simulink model "TwoDSim"  (R2021b)
settings: Solver=VariableStepAuto  StartTime=0.0  StopTime=5  RelTol=1e-3
undefined symbols (not defined in the file): Dterm, Iterm, Pterm
libraries: simulink_extras x5, simulink x1, slpidlib x1
settings Model: Creator=Andres  LastModifiedBy=Andres
settings SolverCC: ZeroCrossAlgorithm=Adaptive
settings DebuggingCC: IgnoredZcDiagnostic=none

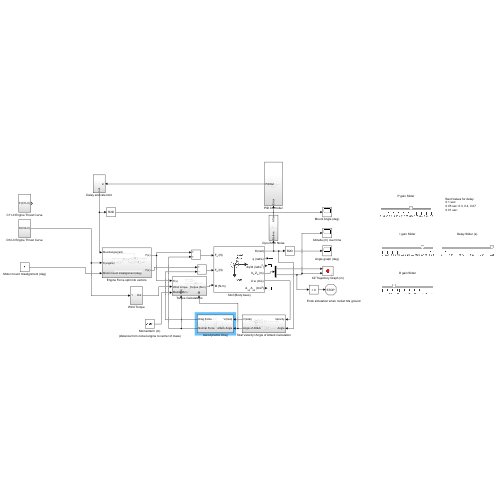
[thumbnail: Simulink's stored preview of the top-level diagram]
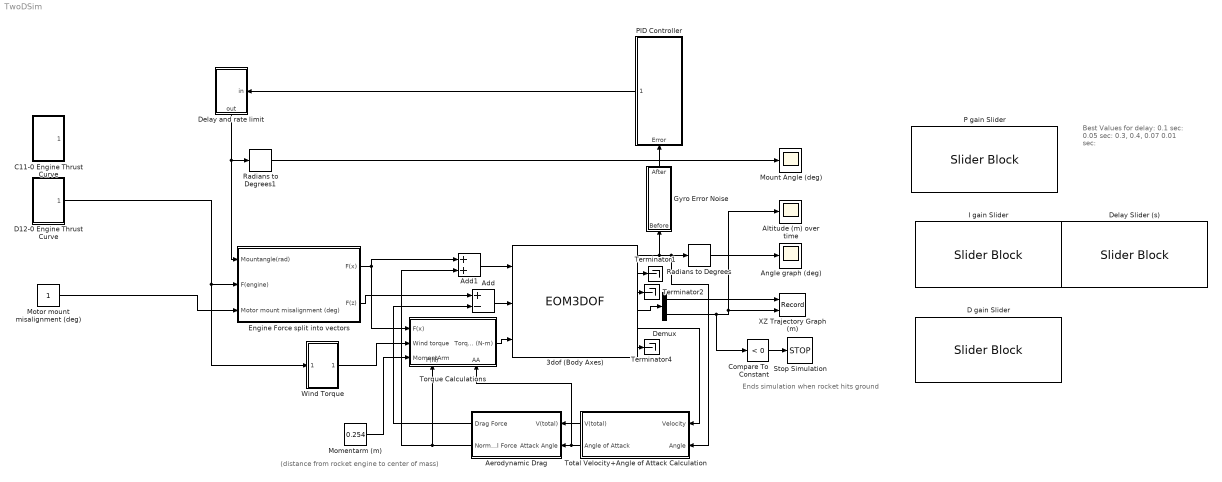
== system TwoDSim ==
  note: Ends simulation when rocket hits ground
  note: (distance from rocket engine to center of mass)
  note: Best Values for delay:
      | 0.1 sec:
      | 0.05 sec: 0.3, 0.4, 0.07
      | 0.01 sec:
  3dof (Body Axes) : EOM3DOF  v_ini=0.00000000000000000001  pos_ini=[0 0.1]  mass=0.688  Iyy=0.012545  g=-9.81
  Add : Sum  Inputs=+-
  Add1 : Sum
  Aerodynamic Drag : Subsystem
  Altitude (m) over time : Scope
  Angle graph (deg) : Scope
  C11-0 Engine Thrust Curve : Subsystem
  Compare To Constant : simulink/Logic and Bit Operations/Compare To Constant  relop=<  const=0  OutDataTypeStr=boolean
  D gain Slider : SliderBlock  LabelPosition=Hide  ScaleMax=0.3
  D12-0 Engine Thrust Curve : Subsystem
  Delay Slider (s) : SliderBlock  LabelPosition=Hide  ScaleMax=0.05  TickInterval=0.01
  Delay and rate limit : Subsystem
      settings: PortSchema="{\"entries\":[{\"content\":{\"sides\":[{\"content\":{\"connectorIds\":[\"In1\"]},\"type\":\"ConnectorPlacement.EquallySpacedRectSide\",\"uuid\":\"7f945310-91d5-4a5b-a152-cb378cea97e0\"},{\"content\":{\"connectorIds\":[],\"side\":\"RIGHT\"},\"type\":\"ConnectorPlacement.EquallySpacedRectSide\",\"uuid\":\"570eb395-808b-402d-8169-834796957515\"},{\"content\":{\"connectorIds\":[],\"side\":\"TOP\"},\"type\":\"ConnectorPlacement.EquallySpacedRectSide\",\"uuid\":\"f414d9f5-06db-41f9-9870-e73b040f5e14\"},{\"content\":{\"connectorIds\":[\"Out1\"],\"side\":\"BOTTOM\"},\"type\":\"ConnectorPlacement.EquallySpacedRectSide\",\"uuid\":\"dd3ad95d-53d5-4309-a4ef-7403eee50954\"}]},\"type\":\"ConnectorPlacement.EquallySpacedConnector\",\"uuid\":\"16f64462-feef-497e-ac9f-2db815891e61\"}],\"packageUris\":[\"http://schema.mathworks.com/mf0/Connector/R2020b\"],\"version\":\"1.0\"}"
  Demux : Demux  Outputs=2
  Engine Force split into vectors : Subsystem
  Gyro Error Noise : Subsystem
      settings: PortSchema="{\"entries\":[{\"content\":{\"sides\":[{\"content\":{\"connectorIds\":[]},\"type\":\"ConnectorPlacement.EquallySpacedRectSide\",\"uuid\":\"db613b74-a95a-4e78-b0b5-852c38ce090d\"},{\"content\":{\"connectorIds\":[],\"side\":\"RIGHT\"},\"type\":\"ConnectorPlacement.EquallySpacedRectSide\",\"uuid\":\"8ff7bb38-cc09-4562-ae4b-2277c61965ca\"},{\"content\":{\"connectorIds\":[\"Out1\"],\"side\":\"TOP\"},\"type\":\"ConnectorPlacement.EquallySpacedRectSide\",\"uuid\":\"fa7b536e-f18b-43ee-b35a-7562f98f0dcc\"},{\"content\":{\"connectorIds\":[\"In1\"],\"side\":\"BOTTOM\"},\"type\":\"ConnectorPlacement.EquallySpacedRectSide\",\"uuid\":\"dd72ef68-23e3-4e8c-8031-36f0d8372741\"}]},\"type\":\"ConnectorPlacement.EquallySpacedConnector\",\"uuid\":\"56970b38-3c02-4837-94fb-dc8b3090c774\"}],\"packageUris\":[\"http://schema.mathworks.com/mf0/Connector/R2020b\"],\"version\":\"1.0\"}"
  I gain Slider : SliderBlock  LabelPosition=Hide  ScaleMax=0.5
  Momentarm (m) : Constant  Value=0.254
  Motor mount misalignment (deg) : Constant
  Mount Angle (deg) : Scope
  P gain Slider : SliderBlock  LabelPosition=Hide  ScaleMax=0.5
  PID Controller : Subsystem
      settings: PortSchema="{\"entries\":[{\"content\":{\"sides\":[{\"content\":{\"connectorIds\":[\"Out1\"]},\"type\":\"ConnectorPlacement.EquallySpacedRectSide\",\"uuid\":\"3056940d-b626-4ad3-aea6-cbabeac63329\"},{\"content\":{\"connectorIds\":[],\"side\":\"RIGHT\"},\"type\":\"ConnectorPlacement.EquallySpacedRectSide\",\"uuid\":\"0510cd9b-8fa4-4f8a-80ec-38231d972233\"},{\"content\":{\"connectorIds\":[],\"side\":\"TOP\"},\"type\":\"ConnectorPlacement.EquallySpacedRectSide\",\"uuid\":\"9c9a70ab-b090-41d6-ac7a-a7598bc3d7a5\"},{\"content\":{\"connectorIds\":[\"In1\"],\"side\":\"BOTTOM\"},\"type\":\"ConnectorPlacement.EquallySpacedRectSide\",\"uuid\":\"76047b82-5909-4180-a207-d443029300af\"}]},\"type\":\"ConnectorPlacement.EquallySpacedConnector\",\"uuid\":\"ba61792f-c506-461f-9738-365393edbd5c\"}],\"packageUris\":[\"http://schema.mathworks.com/mf0/Connector/R2020b\"],\"version\":\"1.0\"}"
  Radians to Degrees : simulink_extras/Transformations/Radians to Degrees
  Radians to Degrees1 : simulink_extras/Transformations/Radians to Degrees
  Stop Simulation : Stop
  Terminator1 : Terminator
  Terminator2 : Terminator
  Terminator4 : Terminator
  Torque Calculations : Subsystem
      settings: PortSchema="{\"entries\":[{\"content\":{\"sides\":[{\"content\":{\"connectorIds\":[\"In1\",\"In2\",\"In3\"]},\"type\":\"ConnectorPlacement.EquallySpacedRectSide\",\"uuid\":\"46c9bf12-68cd-4f09-8bad-0e00413da724\"},{\"content\":{\"connectorIds\":[\"Out1\"],\"side\":\"RIGHT\"},\"type\":\"ConnectorPlacement.EquallySpacedRectSide\",\"uuid\":\"5cb401ed-1243-45d0-bdc5-af7640ec82b5\"},{\"content\":{\"connectorIds\":[],\"side\":\"TOP\"},\"type\":\"ConnectorPlacement.EquallySpacedRectSide\",\"uuid\":\"5f043d3f-b6cd-41df-bbf2-4ec5056a4b50\"},{\"content\":{\"connectorIds\":[\"In4\",\"In5\"],\"side\":\"BOTTOM\"},\"type\":\"ConnectorPlacement.EquallySpacedRectSide\",\"uuid\":\"42e4a957-daef-4922-8ac0-104dea8142f2\"}]},\"type\":\"ConnectorPlacement.EquallySpacedConnector\",\"uuid\":\"e504a0e6-5ad1-4450-ab64-4c7c7eb6b0a6\"}],\"packageUris\":[\"http://schema.mathworks.com/mf0/Connector/R2020b\"],\"version\":\"1.0\"}"
  Total Velocity+Angle of Attack Calculation : Subsystem
  Wind Torque : Subsystem
  XZ Trajectory Graph (m) : Record  FileSettingsInternal="{\"entries\":[{\"content\":{\"excelSettings\":{\"content\":{},\"type\":\"Streamout.ExcelSettings\"}},\"type\":\"Streamout.FileSettingStorage\",\"uuid\":\"bb20e1d7-6d9a-4e8f-a0b6-b3d1b4dfe27c\"}],\"packageUris\":[\"http://schema.mathworks.com/mf0/streamout_blocks/R2020a\"],\"version\":\"1.0\"}"  Layout=[1 1]  SignalsInternal="{\"entries\":[{\"content\":{\"signals\":[{\"content\":{\"blockPath\":[\"TwoDSim/XZ Trajectory Graph (m)\"],\"channel\":[],\"dimensions\":[1],\"domain\":\"TwoDSim/XZ Trajectory Graph (m)\",\"lineColor\":\"#fe330a\",\"plots\":[1],\"port\":1,\"sid\":[\"\"],\"signalID\":2931,\"signalName\":\"Demux:1\"},\"type\":\"RecordBlkView.Signal\",\"uuid\":\"c85508b4-ab53-4732-8bef-55b80f18123d\"},{\"content\":{\"blockPath\":[\"TwoDSim/XZ Trajectory Graph (m)\"],\"channel\":[],\"dimensions\":[1],\"domain\":\"TwoDSim/XZ Trajectory Graph (m)\",\"lineColor\":\"#22b573\",\"plots\":[1],\"port\":2,\"sid\":[\"\"],\"signalID\":2935,\"signalName\":\"Demux:2\"},\"type\":\"RecordBlkView.Signal\",\"uuid\":\"00a216d9-84cc-46e3-ad5b-dcc96f16472e\"}]},\"type\":\"RecordBlkView.InputSignals\",\"uuid\":\"2a0ec8b3-2e71-440f-9c62-95db134db282\"}],\"packageUris\":[\"http://schema.mathworks.com/mf0/streamout_blocks/R2020a\"],\"version\":\"1.0\"}"  VisualizationBindings="{\"xyplotplugin\":{\"info\":[{\"series\":[{\"bindingParametersList\":[{\"parameter\":\"X-Axis\",\"signalID\":2931,\"signalName\":\"Demux:1\"},{\"parameter\":\"Y-Axis\",\"signalID\":2935,\"signalName\":\"Demux:2\"}],\"seriesID\":12514}],\"subplotID\":1}]}}"  CompatibilityTag=XY
  wires:
  3dof (Body Axes)/4 -> Demux/1
  Demux/2 -> Altitude (m) over time/1, XZ Trajectory Graph (m)/2, Compare To Constant/1
  Compare To Constant/1 -> Stop Simulation/1
  Demux/1 -> XZ Trajectory Graph (m)/1
  3dof (Body Axes)/3 -> Terminator2/1
  3dof (Body Axes)/6 -> Terminator4/1
  3dof (Body Axes)/2 -> Terminator1/1
  Motor mount misalignment (deg)/1 -> Engine Force split into vectors/3(Motor mount misalignment (deg))
  Radians to Degrees/1 -> Angle graph (deg)/1
  PID Controller/1(PIDOut) -> Delay and rate limit/1(in)
  3dof (Body Axes)/1 -> Radians to Degrees/1, Total Velocity+Angle of Attack Calculation/2(Angle), Gyro Error Noise/1(Before)
  D12-0 Engine Thrust Curve/1(F(D12-0)) -> Wind Torque/1(Inport), Engine Force split into vectors/2(F(engine))
  Gyro Error Noise/1(After) -> PID Controller/1(Error)
  Delay and rate limit/1(out) -> Radians to Degrees1/1, Engine Force split into vectors/1(Mountangle(rad))
  Wind Torque/1(Out) -> Torque Calculations/2(Wind torque)
  Momentarm (m)/1 -> Torque Calculations/3(MomentArm)
  Radians to Degrees1/1 -> Mount Angle (deg)/1
  Engine Force split into vectors/2(F(z)) -> Add/1
  3dof (Body Axes)/5 -> Total Velocity+Angle of Attack Calculation/1(Velocity)
  Add/1 -> 3dof (Body Axes)/2
  Engine Force split into vectors/1(F(x)) -> Torque Calculations/1(F(x)), Add1/1
  Torque Calculations/1(Torque (N-m)) -> 3dof (Body Axes)/3
  Total Velocity+Angle of Attack Calculation/1(V(total)) -> Aerodynamic Drag/1(V(total))
  Total Velocity+Angle of Attack Calculation/2(Angle of Attack) -> Torque Calculations/5(AA), Aerodynamic Drag/2(Attack Angle)
  Aerodynamic Drag/1(Drag Force) -> Add/2
  Add1/1 -> 3dof (Body Axes)/1
  Aerodynamic Drag/2(Normal Force) -> Torque Calculations/4(F(N)), Add1/2

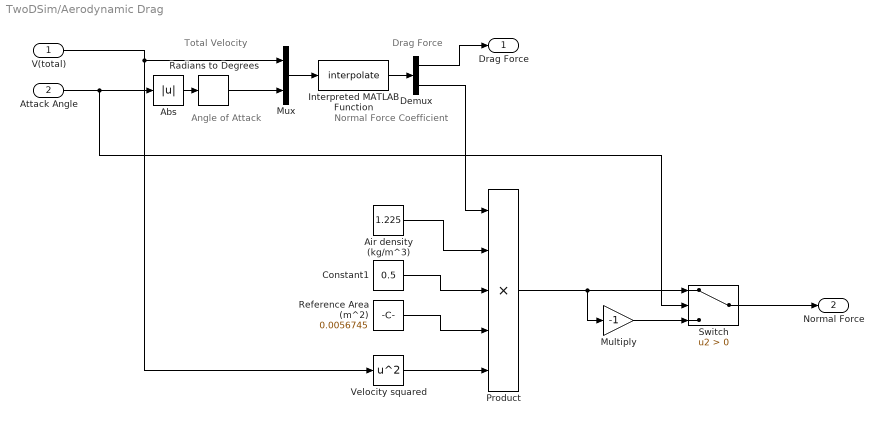
== system TwoDSim/Aerodynamic Drag ==
  note: Normal Force Coefficient
  note: Drag Force
  note: Angle of Attack
  note: Total Velocity
  V(total) : Inport
  Attack Angle : Inport  Port=2
  Abs : Abs
  Air density (kg/m^3) : Constant  Value=1.225
  Constant1 : Constant  Value=0.5
  Demux : Demux  Outputs=2
  Interpreted MATLAB Function : MATLABFcn  MATLABFcn=interpolate
  Multiply : Gain  Gain=-1
  Mux : Mux  Inputs=2
  Product : Product  Inputs=5
  Radians to Degrees : simulink_extras/Transformations/Radians to Degrees
  Reference Area (m^2) : Constant  Value=0.0056745
  Switch : Switch  Criteria=u2 > Threshold
  Velocity squared : Math  Operator=square  SaturateOnIntegerOverflow=on
  Drag Force : Outport
  Normal Force : Outport  Port=2
  wires:
  Attack Angle/1 -> Switch/2, Abs/1
  Air density (kg/m^3)/1 -> Product/2
  Constant1/1 -> Product/3
  Reference Area (m^2)/1 -> Product/4
  Velocity squared/1 -> Product/5
  Abs/1 -> Radians to Degrees/1
  Product/1 -> Multiply/1, Switch/1
  Multiply/1 -> Switch/3
  Switch/1 -> Normal Force/1
  Demux/1 -> Drag Force/1
  Demux/2 -> Product/1
  Interpreted MATLAB Function/1 -> Demux/1
  Mux/1 -> Interpreted MATLAB Function/1
  Radians to Degrees/1 -> Mux/2
  V(total)/1 -> Mux/1, Velocity squared/1

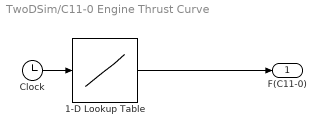
== system TwoDSim/C11-0 Engine Thrust Curve ==
  1-D Lookup Table : Lookup_n-D  NumberOfTableDimensions=1  BreakpointsForDimension1=[0 0.034 0.066 0.107 0.145 0.183 0.214 0.226 0.256 0.281 0.298 0.306 0.323 0.337 0.358 0.385 0.413 0.468 0.539 0.619 0.683 0.715 0.726 0.74 0.758 0.778 0.795 0.81]  Table=[0 1.692 3.782 7.566 10.946 14.832 17.618 18.213 20.107 21.208 21.73 20.206 17.321 14.931 13.236 11.947 11.65 10.946 10.45 10.648 10.648 10.648 10.053 8.163 5.773 3.185 1.394 0]  ExtrapMethod=Clip  InternalRulePriority=Speed  RndMeth=Simplest  InputSameDT=on
  Clock : Clock
  F(C11-0) : Outport
  wires:
  Clock/1 -> 1-D Lookup Table/1
  1-D Lookup Table/1 -> F(C11-0)/1

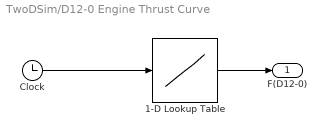
== system TwoDSim/D12-0 Engine Thrust Curve ==
  1-D Lookup Table : Lookup_n-D  NumberOfTableDimensions=1  BreakpointsForDimension1=[0 0.049 0.116 0.184 0.237 0.282 0.297 0.311 0.322 0.348 0.386 0.442 0.546 0.718 0.879 1.066 1.257 1.436 1.59 1.612 1.65]  Table=[0 2.569 9.369 17.275 24.258 29.73 27.01 22.589 17.99 14.126 12.099 10.808 9.876 9.306 9.105 8.901 8.698 8.31 8.294 4.613 0]  ExtrapMethod=Clip  UseLastTableValue=on  InternalRulePriority=Speed  RndMeth=Nearest  InputSameDT=on
  Clock : Clock
  F(D12-0) : Outport
  wires:
  Clock/1 -> 1-D Lookup Table/1
  1-D Lookup Table/1 -> F(D12-0)/1

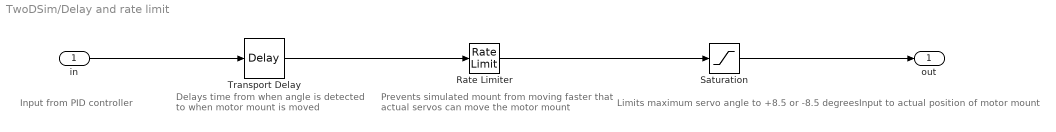
== system TwoDSim/Delay and rate limit ==
  note: Input to actual position of motor mount
  note: Input from PID controller
  note: Limits maximum servo angle to +8.5 or -8.5 degrees
  note: Prevents simulated mount from moving faster
      | that actual servos can move the motor mount
  note: Delays time from when angle is
      | detected to when motor mount is moved
  in : Inport
  Rate Limiter : RateLimiter  RisingSlewLimit=4.5  FallingSlewLimit=-4.5  SampleTimeMode=inherited
  Saturation : Saturate  UpperLimit=0.148353  LowerLimit=-0.148353
  Transport Delay : TransportDelay  DelayTime=0.05
  out : Outport
  wires:
  Transport Delay/1 -> Rate Limiter/1
  in/1 -> Transport Delay/1
  Rate Limiter/1 -> Saturation/1
  Saturation/1 -> out/1

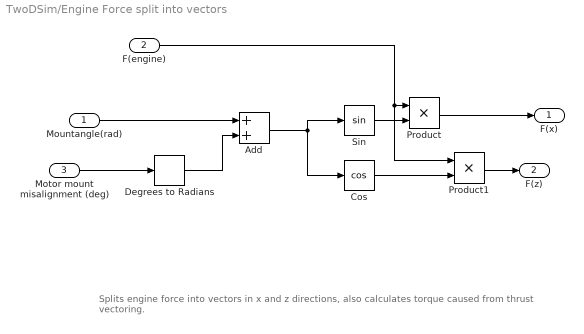
== system TwoDSim/Engine Force split into vectors ==
  note: Splits engine force into vectors in x and z directions, also calculates torque caused from thrust vectoring.
  Mountangle(rad) : Inport
  F(engine) : Inport  Port=2
  Motor mount misalignment (deg) : Inport  Port=3
  Add : Sum
  Cos : Trigonometry  Operator=cos
  Degrees to Radians : simulink_extras/Transformations/Degrees to Radians
  Product : Product
  Product1 : Product
  Sin : Trigonometry
  F(x) : Outport
  F(z) : Outport  Port=2
  wires:
  Sin/1 -> Product/2
  Product1/1 -> F(z)/1
  Cos/1 -> Product1/2
  Product/1 -> F(x)/1
  F(engine)/1 -> Product1/1, Product/1
  Mountangle(rad)/1 -> Add/1
  Add/1 -> Cos/1, Sin/1
  Degrees to Radians/1 -> Add/2
  Motor mount misalignment (deg)/1 -> Degrees to Radians/1

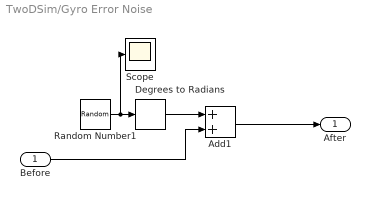
== system TwoDSim/Gyro Error Noise ==
  Before : Inport
  Add1 : Sum
  Degrees to Radians : simulink_extras/Transformations/Degrees to Radians
  Random Number1 : RandomNumber  Variance=0.01  SampleTime=0.1
  Scope : Scope
  After : Outport
  wires:
  Degrees to Radians/1 -> Add1/1
  Before/1 -> Add1/2
  Random Number1/1 -> Scope/1, Degrees to Radians/1
  Add1/1 -> After/1

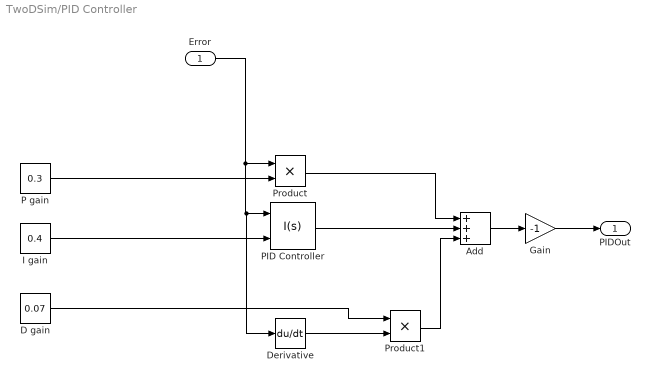
== system TwoDSim/PID Controller ==
  Error : Inport
  Add : Sum  Inputs=+++
  D gain : Constant  Value=0.07
  Derivative : Derivative
  Gain : Gain  Gain=-1
  I gain : Constant  Value=0.4
  P gain : Constant  Value=0.3
  PID Controller : slpidlib/PID Controller  Controller=I  Form=Parallel  TimeDomain=Continuous-time  UseExternalTs=off  SampleTime=-1  IntegratorMethod=Forward Euler  FilterMethod=Forward Euler  ControllerParametersSource=external  P=Pterm  I=Iterm  D=Dterm  UseFilter=on  N=100  TunerSelectOption=Transfer Function Based (PID Tuner App)  InitialConditionSource=internal  InitialConditionForIntegrator=0  InitialConditionForFilter=0  DifferentiatorICPrevScaledInput=0  ExternalReset=none  TrackingMode=off  Kt=1  LimitOutput=off  SatLimitsSource=internal  UpperSaturationLimit=inf  LowerSaturationLimit=-inf  LinearizeAsGain=on  AntiWindupMode=none  Kb=1  POutMin=[]  POutMax=[]  IOutMin=[]  IOutMax=[]  DOutMin=[]  DOutMax=[]  NOutMin=[]  NOutMax=[]  SumOutMin=[]  SumOutMax=[]  SaturationOutMin=[]  SaturationOutMax=[]  PParamMin=[]  PParamMax=[]  IParamMin=[]  IParamMax=[]  DParamMin=[]  DParamMax=[]  NParamMin=[]  NParamMax=[]  KbParamMin=[]  KbParamMax=[]  KtParamMin=[]  KtParamMax=[]  KbOutMin=[]  KbOutMax=[]  KtOutMin=[]  KtOutMax=[]  IntegratorOutMin=[]  IntegratorOutMax=[]  FilterOutMin=[]  FilterOutMax=[]  SumI1OutMin=[]  SumI1OutMax=[]  SumI2OutMin=[]  SumI2OutMax=[]  SumI3OutMin=[]  SumI3OutMax=[]  SumI4OutMin=[]  SumI4OutMax=[]  SumDOutMin=[]  SumDOutMax=[]  DifferentiatorOutMin=[]  DifferentiatorOutMax=[]  FilterDiffOutCoefMin=[]  FilterDiffOutCoefMax=[]  ReciprocalOutMin=[]  ReciprocalOutMax=[]  SumDenOutMin=[]  SumDenOutMax=[]  SumNumOutMin=[]  SumNumOutMax=[]  DivideOutMin=[]  DivideOutMax=[]  UdiffTsProdOutMin=[]  UdiffTsProdOutMax=[]  NTsProdOutMin=[]  NTsProdOutMax=[]  UintegralTsProdOutMin=[]  UintegralTsProdOutMax=[]  UngainTsProdOutMin=[]  UngainTsProdOutMax=[]  IntegratorContinuousStateAttributes=''  IntegratorStateMustResolveToSignalObject=off  IntegratorRTWStateStorageClass=Auto  FilterContinuousStateAttributes=''  FilterStateMustResolveToSignalObject=off  FilterRTWStateStorageClass=Auto  ParallelPVariant=Disabled  IdealPVariant=Disabled  IVariant=ExternalParameters  DVariant=Disabled  IntegratorVariant=Continuous  SatVariant=Disabled  AWVariant=Passthrough  PCopyVariant=Disabled  TRVariant=Disabled  FdbkBlocksVariant=Forward  IdealPFdbkVariant=Disabled  SatFdbkVariant=Disabled  DerivativeFilterVariant=Disabled  NVariant=Disabled  NCopyVariant=Disabled_SignalSpec  FilterICVariant=Disabled  IntegratorICVariant=InternalICs  ExternalResetVariant=Disabled  TRSumVariant=Passthrough  SumFdbkVariant=Disabled  SumVariant=Passthrough_I  TsampFilterVariant=InternalTs  TsampNgainVariant=Passthrough  TsampIntegralVariant=Passthrough  ExternalSaturationOutDataTypeStr=Inherit: Same as second input
  Product : Product
  Product1 : Product
  PIDOut : Outport
  wires:
  Error/1 -> Derivative/1, PID Controller/1, Product/1
  Gain/1 -> PIDOut/1
  Add/1 -> Gain/1
  Product/1 -> Add/1
  PID Controller/1 -> Add/2
  P gain/1 -> Product/2
  Derivative/1 -> Product1/2
  Product1/1 -> Add/3
  I gain/1 -> PID Controller/2
  D gain/1 -> Product1/1

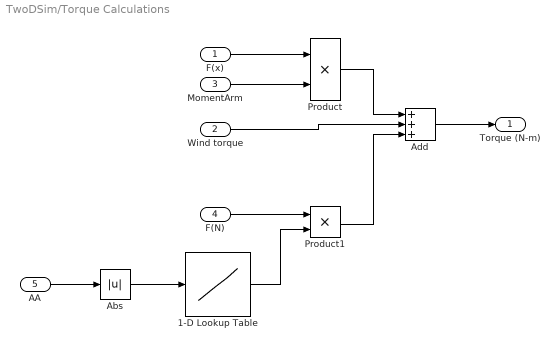
== system TwoDSim/Torque Calculations ==
  F(x) : Inport
  Wind torque : Inport  Port=2
  MomentArm : Inport  Port=3
  F(N) : Inport  Port=4
  AA : Inport  Port=5
  1-D Lookup Table : Lookup_n-D  NumberOfTableDimensions=1  BreakpointsForDimension1=|  Table=|  InternalRulePriority=Speed  RndMeth=Simplest  InputSameDT=on
      BreakpointsForDimension1=|
      | [0
      | 5
      | 10
      | 15
      | 20
      | 25
      | 30
      | 35
      | 40
      | 45
      | 50
      | 55
      | 60
      | 65
      | 70
      | 75
      | 80
      | 85
      | 90
      | 95
      | 100
      | 105
      | 110
      | 115
      | 120
      | 125
      | 130
      | 135
      | 140
      | 145
      | 150
      | 155
      | 160
      | 165
      | 170
      | 175
      | 180]
      Table=|
      | [31.84
      | 24.9
      | 21
      | 18.6
      | 16.9
      | 15.7
      | 14.8
      | 14
      | 13.5
      | 13.1
      | 12.7
      | 12.4
      | 12.2
      | 12
      | 11.9
      | 11.8
      | 11.7
      | 11.6
      | 11.6
      | 11.6
      | 11.7
      | 11.8
      | 11.9
      | 12
      | 12.2
      | 12.4
      | 12.7
      | 13.1
      | 13.5
      | 14
      | 14.8
      | 15.7
      | 1.69E+01
      | 1.86E+01
      | 21
      | 24.9
      | 31.84]
  Abs : Abs
  Add : Sum  Inputs=+++
  Product : Product
  Product1 : Product
  Torque (N-m) : Outport
  wires:
  Add/1 -> Torque (N-m)/1
  F(x)/1 -> Product/1
  MomentArm/1 -> Product/2
  Product/1 -> Add/1
  Wind torque/1 -> Add/2
  F(N)/1 -> Product1/1
  1-D Lookup Table/1 -> Product1/2
  Product1/1 -> Add/3
  AA/1 -> Abs/1
  Abs/1 -> 1-D Lookup Table/1

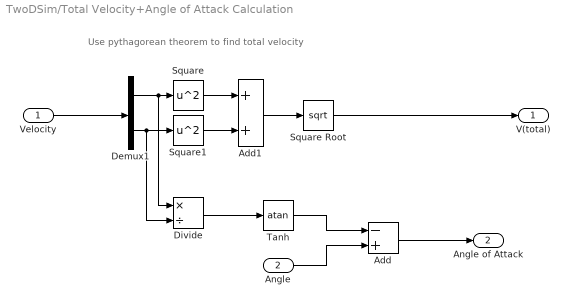
== system TwoDSim/Total Velocity+Angle of Attack Calculation ==
  note: Use pythagorean theorem to find total velocity
  Velocity : Inport
  Angle : Inport  Port=2
  Add : Sum  Inputs=-+
  Add1 : Sum
  Demux1 : Demux  Outputs=2
  Divide : Product  Inputs=*/
  Square : Math  Operator=square  SaturateOnIntegerOverflow=on
  Square Root : Sqrt  SaturateOnIntegerOverflow=on
  Square1 : Math  Operator=square  SaturateOnIntegerOverflow=on
  Tanh : Trigonometry  Operator=atan
  V(total) : Outport
  Angle of Attack : Outport  Port=2
  wires:
  Square1/1 -> Add1/2
  Demux1/2 -> Divide/2, Square1/1
  Demux1/1 -> Divide/1, Square/1
  Velocity/1 -> Demux1/1
  Square Root/1 -> V(total)/1
  Add1/1 -> Square Root/1
  Square/1 -> Add1/1
  Divide/1 -> Tanh/1
  Tanh/1 -> Add/1
  Angle/1 -> Add/2
  Add/1 -> Angle of Attack/1

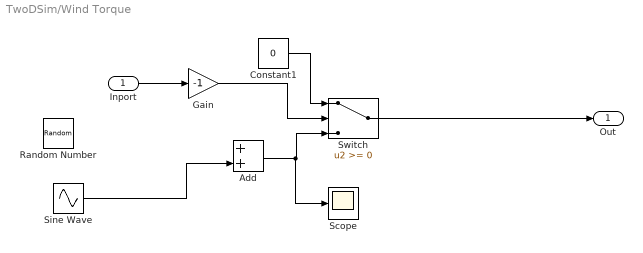
== system TwoDSim/Wind Torque ==
  Inport : Inport
  Add : Sum
  Constant1 : Constant  Value=0
  Gain : Gain  Gain=-1
  Random Number : RandomNumber  Variance=0.00005  Seed=5  SampleTime=0.1
  Scope : Scope
  Sine Wave : Sin  Amplitude=0.05  Bias=0.15  Frequency=2.5  SampleTime=0
  Switch : Switch
  Out : Outport
  wires:
  Constant1/1 -> Switch/1
  Gain/1 -> Switch/2
  Inport/1 -> Gain/1
  Switch/1 -> Out/1
  Add/1 -> Scope/1, Switch/3
  Sine Wave/1 -> Add/2
